simulink model "BLDC"  (R2024b)
settings: Solver=VariableStepAuto  StartTime=0.0  StopTime=10  RelTol=1e-3
values from neighbouring files (symbols this model uses):
  b_eq = b_l*(1/r)^2+b_m    (= 2.36823386114e-05)    [Parametros.m]
  J_eq = J_l*(1/r)^2+J_m    [Parametros.m]
  K_e = 0.0217    [Parametros.m]
  k_l = m*g*l_cm+m_l*g*l_l    [Parametros.m]
  L_s = 0.113e-3    (= 0.000113)    [Parametros.m]
  p = 7    [Parametros.m]
  psi_m = K_e/(1.5*p)    (= 0.00206666666667)    [Parametros.m]
  r = 156    [Parametros.m]
  R_s = 0.196    [Parametros.m]
  U_d = 18    [Parametros.m]
libraries: eePwmGenerator x1, simulink x1
settings Model: Creator=ribei  LastModifiedBy=ribei

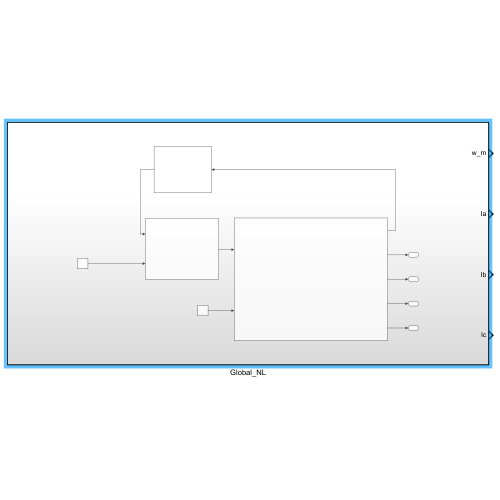
[thumbnail: Simulink's stored preview of the top-level diagram]
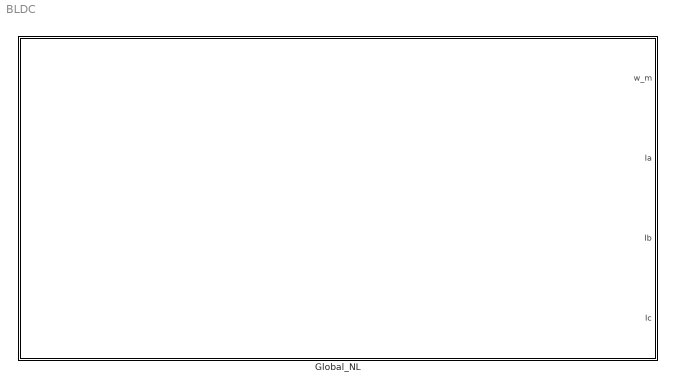
== system BLDC ==
  Global_NL : Subsystem

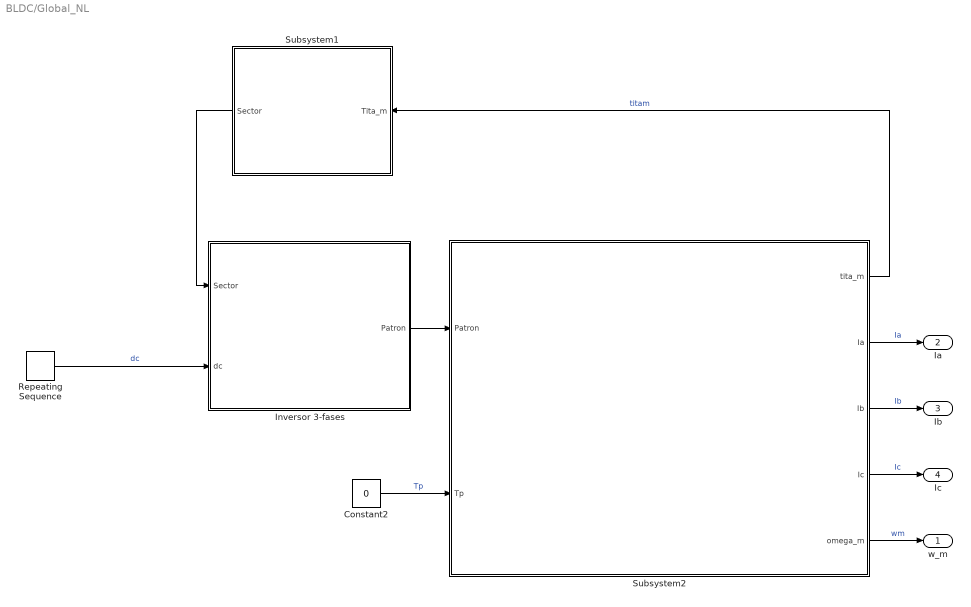
== system BLDC/Global_NL ==
  Constant2 : Constant  Value=0
  Inversor 3-fases : Subsystem
  Repeating Sequence : simulink/Sources/Repeating Sequence  rep_seq_t=[0 2 4 6 8 10]  rep_seq_y=[0 0.25 0.25 0.5 0.5 0.75]
  Subsystem1 : Subsystem
  Subsystem2 : Subsystem
  w_m : Outport
  Ia : Outport  Port=2
  Ib : Outport  Port=3
  Ic : Outport  Port=4
  wires:
  Subsystem1/1(Sector) -> Inversor 3-fases/1(Sector)
  Inversor 3-fases/1(Patron) -> Subsystem2/1(Patron)
  Subsystem2/1(tita_m) -> Subsystem1/1(Tita_m)  "titam"
  Subsystem2/2(Ia) -> Ia/1  "Ia"
  Subsystem2/3(Ib) -> Ib/1  "Ib"
  Subsystem2/4(Ic) -> Ic/1  "Ic"
  Subsystem2/5(omega_m) -> w_m/1  "wm"
  Constant2/1 -> Subsystem2/2(Tp)  "Tp"
  Repeating Sequence/1 -> Inversor 3-fases/2(dc)  "dc"

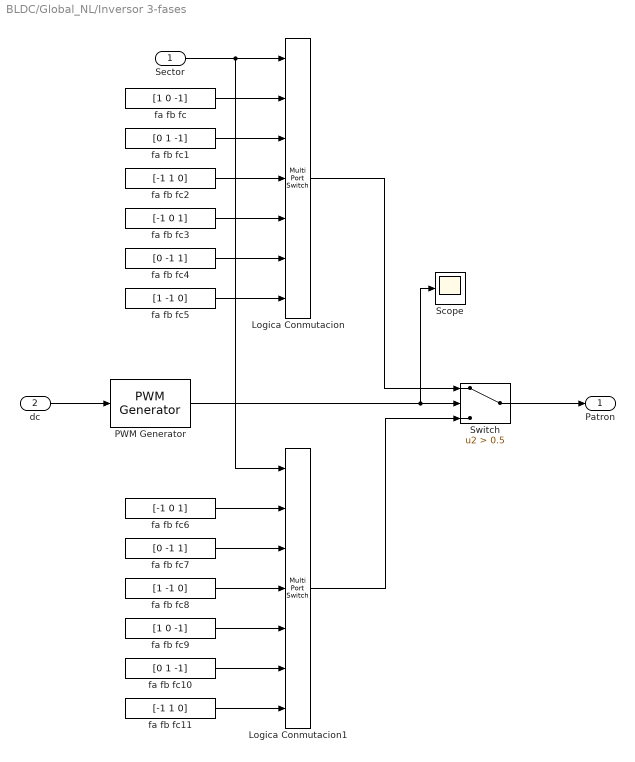
== system BLDC/Global_NL/Inversor 3-fases ==
  Sector : Inport
  dc : Inport  Port=2
  Logica Conmutacion : MultiPortSwitch  Inputs=6  DiagnosticForDefault=None  SaturateOnIntegerOverflow=off  InputSameDT=off
  Logica Conmutacion1 : MultiPortSwitch  Inputs=6  DiagnosticForDefault=None  SaturateOnIntegerOverflow=off  InputSameDT=off
  PWM Generator : eePwmGenerator/PWM Generator  CarrCount=Up  Tper=0.001  Tdelay=0  Ts=5e-5
  Scope : Scope
  Switch : Switch  Criteria=u2 > Threshold  Threshold=0.5  SaturateOnIntegerOverflow=off  InputSameDT=off
  fa fb fc : Constant  Value=[1 0 -1]
  fa fb fc1 : Constant  Value=[0 1 -1]
  fa fb fc10 : Constant  Value=[0 1 -1]
  fa fb fc11 : Constant  Value=[-1 1 0]
  fa fb fc2 : Constant  Value=[-1 1 0]
  fa fb fc3 : Constant  Value=[-1 0 1]
  fa fb fc4 : Constant  Value=[0 -1 1]
  fa fb fc5 : Constant  Value=[1 -1 0]
  fa fb fc6 : Constant  Value=[-1 0 1]
  fa fb fc7 : Constant  Value=[0 -1 1]
  fa fb fc8 : Constant  Value=[1 -1 0]
  fa fb fc9 : Constant  Value=[1 0 -1]
  Patron : Outport
  wires:
  Switch/1 -> Patron/1
  fa fb fc2/1 -> Logica Conmutacion/4
  fa fb fc5/1 -> Logica Conmutacion/7
  Sector/1 -> Logica Conmutacion/1, Logica Conmutacion1/1
  fa fb fc3/1 -> Logica Conmutacion/5
  fa fb fc4/1 -> Logica Conmutacion/6
  fa fb fc1/1 -> Logica Conmutacion/3
  fa fb fc/1 -> Logica Conmutacion/2
  Logica Conmutacion/1 -> Switch/1
  Logica Conmutacion1/1 -> Switch/3
  fa fb fc9/1 -> Logica Conmutacion1/5
  fa fb fc10/1 -> Logica Conmutacion1/6
  fa fb fc11/1 -> Logica Conmutacion1/7
  fa fb fc7/1 -> Logica Conmutacion1/3
  fa fb fc8/1 -> Logica Conmutacion1/4
  fa fb fc6/1 -> Logica Conmutacion1/2
  PWM Generator/1 -> Scope/1, Switch/2
  dc/1 -> PWM Generator/1

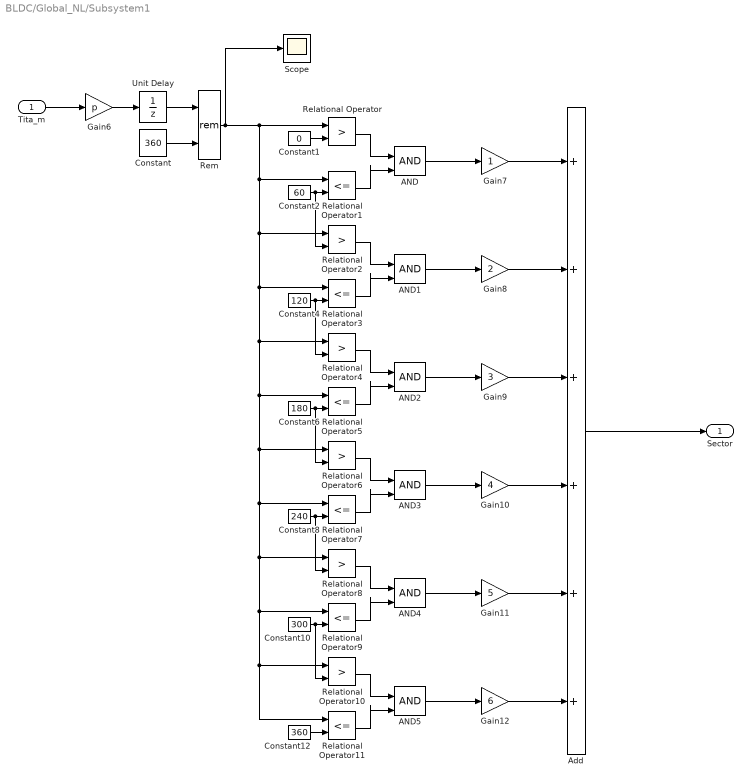
== system BLDC/Global_NL/Subsystem1 ==
  Tita_m : Inport
  AND{,1..5} (6 alike) : Logic  IconShape=distinctive  AllPortsSameDT=off  OutDataTypeStr=boolean
  Add : Sum  Inputs=++++++
  Constant : Constant  Value=360
  Constant1 : Constant  Value=0
  Constant10 : Constant  Value=300
  Constant12 : Constant  Value=360
  Constant2 : Constant  Value=60
  Constant4 : Constant  Value=120
  Constant6 : Constant  Value=180
  Constant8 : Constant  Value=240
  Gain10 : Gain  Gain=4
  Gain11 : Gain  Gain=5
  Gain12 : Gain  Gain=6
  Gain6 : Gain  Gain=p
  Gain7 : Gain
  Gain8 : Gain  Gain=2
  Gain9 : Gain  Gain=3
  Relational Operator{,2,4,6,8,10} (6 alike) : RelationalOperator  Operator=>  OutDataTypeStr=boolean  RndMeth=Simplest  InputSameDT=off
  Relational Operator{1,3,5,7,9,11} (6 alike) : RelationalOperator  Operator=<=  OutDataTypeStr=boolean  RndMeth=Simplest  InputSameDT=off
  Rem : Math  Operator=rem
  Scope : Scope
  Unit Delay : UnitDelay  SampleTime=0.001  HasFrameUpgradeWarning=on
  Sector : Outport
  wires:
  Rem/1 -> Scope/1, Relational Operator/1, Relational Operator1/1, Relational Operator2/1, Relational Operator3/1, Relational Operator4/1, Relational Operator5/1, Relational Operator6/1, Relational Operator7/1, Relational Operator8/1, Relational Operator9/1, Relational Operator10/1, Relational Operator11/1
  AND4/1 -> Gain11/1
  AND1/1 -> Gain8/1
  Relational Operator4/1 -> AND2/1
  Add/1 -> Sector/1
  Gain10/1 -> Add/4
  Relational Operator8/1 -> AND4/1
  Relational Operator3/1 -> AND1/2
  Relational Operator2/1 -> AND1/1
  Gain9/1 -> Add/3
  Constant4/1 -> Relational Operator4/2, Relational Operator3/2
  Constant6/1 -> Relational Operator6/2, Relational Operator5/2
  Gain11/1 -> Add/5
  Constant2/1 -> Relational Operator2/2, Relational Operator1/2
  AND2/1 -> Gain9/1
  Gain7/1 -> Add/1
  Relational Operator5/1 -> AND2/2
  Constant10/1 -> Relational Operator10/2, Relational Operator9/2
  AND/1 -> Gain7/1
  Constant1/1 -> Relational Operator/2
  Relational Operator/1 -> AND/1
  Constant/1 -> Rem/2
  Relational Operator11/1 -> AND5/2
  Constant12/1 -> Relational Operator11/2
  Relational Operator10/1 -> AND5/1
  AND5/1 -> Gain12/1
  Relational Operator9/1 -> AND4/2
  Unit Delay/1 -> Rem/1
  Gain12/1 -> Add/6
  Gain6/1 -> Unit Delay/1
  Tita_m/1 -> Gain6/1
  Constant8/1 -> Relational Operator8/2, Relational Operator7/2
  Relational Operator1/1 -> AND/2
  Relational Operator7/1 -> AND3/2
  AND3/1 -> Gain10/1
  Relational Operator6/1 -> AND3/1
  Gain8/1 -> Add/2

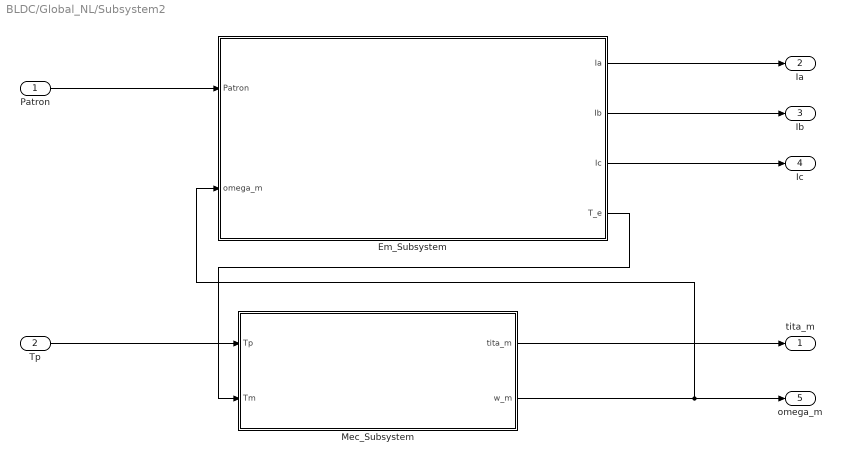
== system BLDC/Global_NL/Subsystem2 ==
  Patron : Inport
  Tp : Inport  Port=2
  Em_Subsystem : Subsystem
  Mec_Subsystem : Subsystem
  tita_m : Outport
  Ia : Outport  Port=2
  Ib : Outport  Port=3
  Ic : Outport  Port=4
  omega_m : Outport  Port=5
  wires:
  Mec_Subsystem/1(tita_m) -> tita_m/1
  Patron/1 -> Em_Subsystem/1(Patron)
  Mec_Subsystem/2(w_m) -> omega_m/1, Em_Subsystem/2(omega_m)
  Em_Subsystem/4(T_e) -> Mec_Subsystem/2(Tm)
  Tp/1 -> Mec_Subsystem/1(Tp)
  Em_Subsystem/1(Ia) -> Ia/1
  Em_Subsystem/3(Ic) -> Ic/1
  Em_Subsystem/2(Ib) -> Ib/1

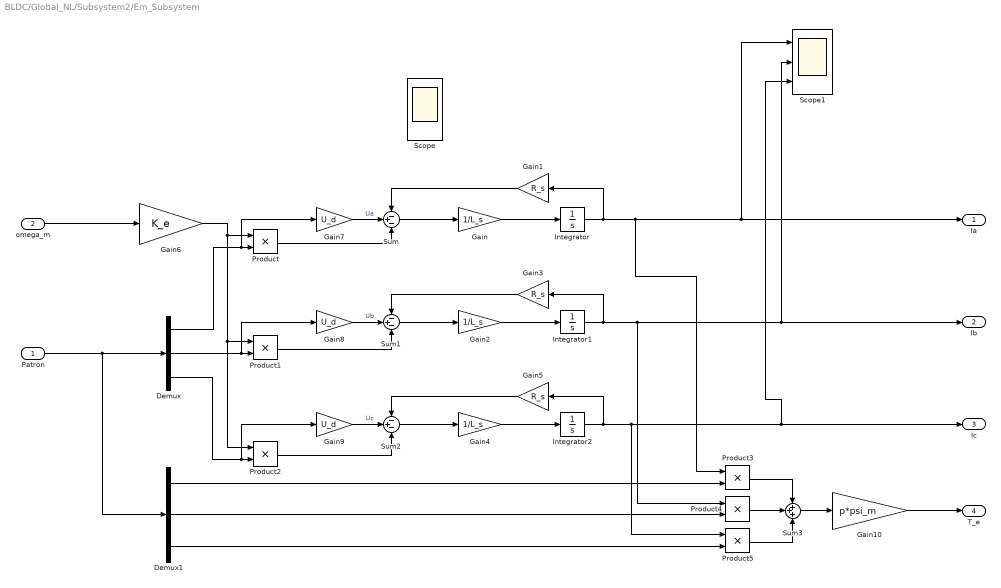
== system BLDC/Global_NL/Subsystem2/Em_Subsystem ==
  Patron : Inport
  omega_m : Inport  Port=2
  Demux : Demux  Outputs=3
  Demux1 : Demux  Outputs=3
  Gain : Gain  Gain=1/L_s
  Gain1 : Gain  Gain=R_s
  Gain10 : Gain  Gain=p*psi_m
  Gain2 : Gain  Gain=1/L_s
  Gain3 : Gain  Gain=R_s
  Gain4 : Gain  Gain=1/L_s
  Gain5 : Gain  Gain=R_s
  Gain6 : Gain  Gain=K_e
  Gain7 : Gain  Gain=U_d
  Gain8 : Gain  Gain=U_d
  Gain9 : Gain  Gain=U_d
  Integrator : Integrator
  Integrator1 : Integrator
  Integrator2 : Integrator
  Product{,1..5} (6 alike) : Product
  Scope : Scope  NumInputPorts=3
  Scope1 : Scope  NumInputPorts=3
  Sum : Sum  Inputs=-+-
  Sum1 : Sum  Inputs=-+-
  Sum2 : Sum  Inputs=-+-
  Sum3 : Sum  Inputs=+++
  Ia : Outport
  Ib : Outport  Port=2
  Ic : Outport  Port=3
  T_e : Outport  Port=4
  wires:
  Gain/1 -> Integrator/1
  Integrator/1 -> Gain1/1, Product3/1, Scope1/1, Ia/1
  Sum/1 -> Gain/1
  Gain1/1 -> Sum/1
  Sum1/1 -> Gain2/1
  Gain3/1 -> Sum1/1
  Gain2/1 -> Integrator1/1
  Integrator1/1 -> Product4/1, Scope1/2, Ib/1, Gain3/1
  Gain4/1 -> Integrator2/1
  Gain5/1 -> Sum2/1
  Sum2/1 -> Gain4/1
  Integrator2/1 -> Product5/1, Scope1/3, Ic/1, Gain5/1
  omega_m/1 -> Gain6/1
  Gain6/1 -> Product2/1, Product1/1, Product/1
  Demux/1 -> Gain7/1, Product/2
  Demux/2 -> Gain8/1, Product1/2
  Demux/3 -> Gain9/1, Product2/2
  Product/1 -> Sum/3
  Product1/1 -> Sum1/3
  Product2/1 -> Sum2/3
  Gain7/1 -> Sum/2  "Ua"
  Gain8/1 -> Sum1/2  "Ub"
  Gain9/1 -> Sum2/2  "Uc"
  Patron/1 -> Demux1/1, Demux/1
  Demux1/1 -> Product3/2
  Demux1/2 -> Product4/2
  Demux1/3 -> Product5/2
  Product3/1 -> Sum3/1
  Product4/1 -> Sum3/2
  Product5/1 -> Sum3/3
  Sum3/1 -> Gain10/1
  Gain10/1 -> T_e/1

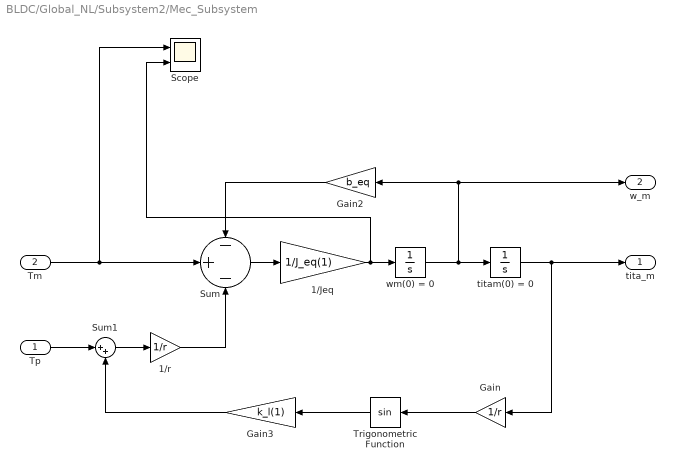
== system BLDC/Global_NL/Subsystem2/Mec_Subsystem ==
  Tp : Inport
  Tm : Inport  Port=2
  1/Jeq : Gain  Gain=1/J_eq(1)
  1/r : Gain  Gain=1/r
  Gain : Gain  Gain=1/r
  Gain2 : Gain  Gain=b_eq
  Gain3 : Gain  Gain=k_l(1)
  Scope : Scope  NumInputPorts=2
  Sum : Sum  Inputs=-+-
  Sum1 : Sum  Inputs=|++
  Trigonometric Function : Trigonometry
  titam(0) = 0 : Integrator
  wm(0) = 0 : Integrator
  tita_m : Outport
  w_m : Outport  Port=2
  wires:
  wm(0) = 0/1 -> Gain2/1, w_m/1, titam(0) = 0/1
  1/r/1 -> Sum/3
  titam(0) = 0/1 -> Gain/1, tita_m/1
  Tp/1 -> Sum1/1
  Sum1/1 -> 1/r/1
  Tm/1 -> Scope/1, Sum/2
  Gain2/1 -> Sum/1
  Sum/1 -> 1/Jeq/1
  Trigonometric Function/1 -> Gain3/1
  1/Jeq/1 -> Scope/2, wm(0) = 0/1
  Gain/1 -> Trigonometric Function/1
  Gain3/1 -> Sum1/2
